simulink model "HelicopterModelingSimulation"  (R2025a)
settings: Solver=FixedStepAuto  StartTime=0.0  StopTime=170  FixedStep=0.01  MaxStep=0.001  RelTol=1e-2
PreLoadFcn:
  | state = "path";
  | visual3D = true;
  | lookDistance = 500;
  | kappa = 0.1;
  | hRef = 20;
  | VRef = 30;
  | WP(:,1) = [0  0  -20]';
  | WP(:,2) = [1500  0  -20]';
  | WP(:,3) = [1500  1000 -20]';
  | WP(:,4) = [0  1000  -20]';
  | WP(:,5) = [0  0  -20]';
model workspace (MAT data in the model file):
  L1 = 3.13
undefined symbols (not defined in the file): gravity, m, rad, rho, s, WP
libraries: slpidlib x9, aerolibconvert2 x5, simulink x3, simulink_extras x3, matrix_library x2, aerolibsim3d x2, aerolibatmos2 x1, aerolibobsolete x1, aerolibasang x1, sim3dlib x1
(part 1 of 4)
settings Model: Creator=The MathWorks, Inc.  LastModifiedBy=2125
settings SolverCC: ZeroCrossAlgorithm=Adaptive
settings DebuggingCC: MaskedZcDiagnostic=none  IgnoredZcDiagnostic=none

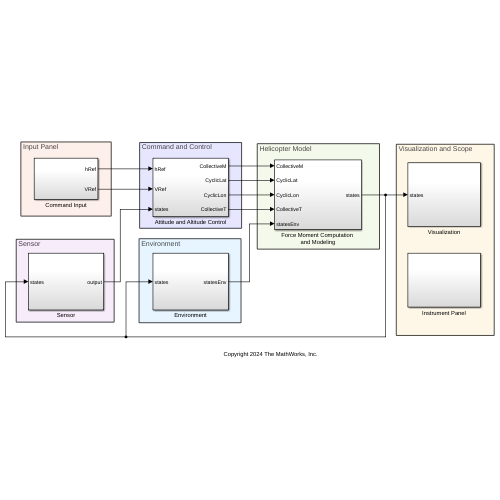
[thumbnail: Simulink's stored preview of the top-level diagram]
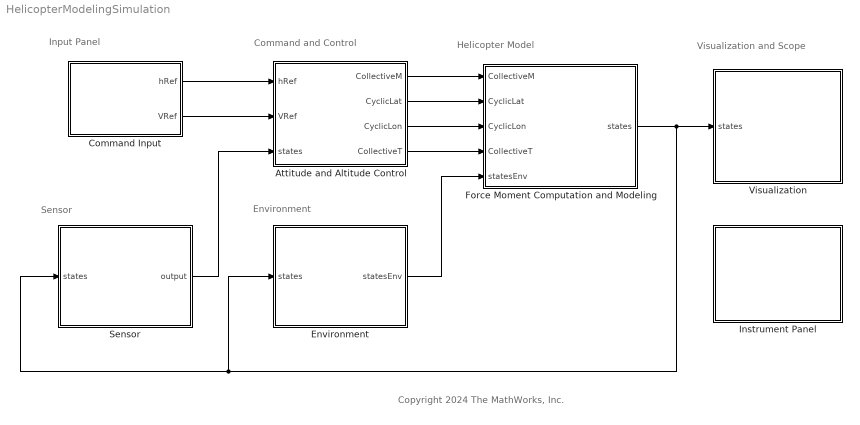
== system HelicopterModelingSimulation ==
  note: Sensor
  note: Input Panel
  note: Copyright 2024 The MathWorks, Inc.
  note: Visualization and Scope
  note: Helicopter Model
  note: Environment
  note: Command and Control
  Attitude and Altitude Control : Subsystem
  Command Input : Subsystem
  Environment : Subsystem
  Force Moment Computation and Modeling : Subsystem
  Instrument Panel : Subsystem
  Sensor : Subsystem
  Visualization : Subsystem
  wires:
  Attitude and Altitude Control/1(CollectiveM) -> Force Moment Computation and Modeling/1(CollectiveM)
  Attitude and Altitude Control/2(CyclicLat) -> Force Moment Computation and Modeling/2(CyclicLat)
  Attitude and Altitude Control/3(CyclicLon) -> Force Moment Computation and Modeling/3(CyclicLon)
  Attitude and Altitude Control/4(CollectiveT) -> Force Moment Computation and Modeling/4(CollectiveT)
  Environment/1(statesEnv) -> Force Moment Computation and Modeling/5(statesEnv)
  Force Moment Computation and Modeling/1(states) -> Sensor/1(states), Environment/1(states), Visualization/1(states)
  Command Input/1(hRef) -> Attitude and Altitude Control/1(hRef)
  Command Input/2(VRef) -> Attitude and Altitude Control/2(VRef)
  Sensor/1(output) -> Attitude and Altitude Control/3(states)

== system HelicopterModelingSimulation/Attitude and Altitude Control ==
  hRef : Inport
  VRef : Inport  Port=2
  states : Inport  Port=3
  Altitude and Attitude Control : Subsystem
  Bus Selector : BusSelector  OutputSignals=Vb,wb,Xe,angles
  Reference Atttiude and Altitude Definition : Subsystem
  CollectiveM : Outport
  CyclicLat : Outport  Port=2
  CyclicLon : Outport  Port=3
  CollectiveT : Outport  Port=4
  wires:
  Reference Atttiude and Altitude Definition/1(posZRef) -> Altitude and Attitude Control/1(posZRef)
  Reference Atttiude and Altitude Definition/2(thetaRef) -> Altitude and Attitude Control/2(thetaRef)
  Altitude and Attitude Control/1(CollectiveM) -> CollectiveM/1
  Reference Atttiude and Altitude Definition/3(phiRef) -> Altitude and Attitude Control/3(phiRef)
  Reference Atttiude and Altitude Definition/4(psiRef) -> Altitude and Attitude Control/4(psiRef)
  Altitude and Attitude Control/3(CyclicLon) -> CyclicLon/1
  Altitude and Attitude Control/4(CollectiveT) -> CollectiveT/1
  Altitude and Attitude Control/2(CyclicLat) -> CyclicLat/1
  Bus Selector/2 -> Altitude and Attitude Control/5(p q r)  "<wb>"
  Bus Selector/4 -> Altitude and Attitude Control/7(angle)  "<angles>"
  Bus Selector/3 -> Reference Atttiude and Altitude Definition/4(Xe), Altitude and Attitude Control/6(Xe)  "<Xe>"
  states/1 -> Bus Selector/1
  Bus Selector/1 -> Reference Atttiude and Altitude Definition/3(Vb)  "<Vb>"
  hRef/1 -> Reference Atttiude and Altitude Definition/1(hRef)
  VRef/1 -> Reference Atttiude and Altitude Definition/2(VRef)
